simulink model "vippattern"  (R2015b)
settings: Solver=FixedStepDiscrete  SolverMode=SingleTasking  StartTime=0.0  StopTime=inf  RelTol=1e-3
InitFcn:
  | % load and initialize the data required by vippattern demo
  | 
  | % get path to the model
  | param_path = 'vippattern/Parameters';
  | 
  | % NOTE:  to set a new target run this command from command prompt:
  | % set_param(param_path,'target',mat2str(target_img))
  | % here, target_img must be a uint8 image
  | 
  | % get AVI file name straight from From MM File block
  | fmmf_path = 'vippattern/From Multimedia File';
  | 
  | % get target which is stored in a hidden parameter of 'Edit Parameters'
  | % subsystem
  | target_img = uint8(eval(get_param(param_path,'target')));
  | 
  | % Create a pyramiding factor variable and initialize it.
  | % Set the pyramiding factor by grabbing it from the masked block
  | % called 'Edit Parameters'
  | pfactor = str2double(get_param(param_path,'pfactor'));
  | 
  | target_dim_nopyramid = size(target_img);
  | % dims for gaussian pyramid
  | target_dim = ceil(target_dim_nopyramid/(2^pfactor));
  | video_info = dspmmfileinfo(get_param(fmmf_path,'inputFilename'));
  | iut_dim = ceil([video_info.videoHeightInPixels video_info.videoWidthInPixels]/2^(pfactor));
  | 
  | % figure out the sizes after padding; padding is necessary in order
  | % to avoid circular convolution
  | target_pad_rows = 2^nextpow2(iut_dim(1)+target_dim(1)+1);
  | target_pad_cols = 2^nextpow2(iut_dim(2)+target_dim(2)+1);
  | 
  | % number of targets to detect (targets are assumed to be identical)
  | num_targets = str2double(get_param(param_path,'num_targets'));
undefined symbols (not defined in the file or in its folder): gray, hot
libraries: visiontransforms x5, visionsinks x3, visionutilities x2, visionstatistics x2, dspvision x1, visiontextngfix x1, vipmisc x1, visiongeotforms x1, visionfilter x1
CloseFcn:
  | clear video_info;
  | clear iut_dim;
  | clear param_path;
  | clear fmmf_path;
  | clear pfactor;
  | clear target_dim;
  | clear target_dim_nopyramid;
  | clear target_img;
  | clear target_pad_cols;
  | clear target_pad_rows;
  | clear num_targets;
settings Model: FPTRunName=Active  ExtModeAutoUpdateStatusClock=off  Creator=The MathWorks, Inc.  LastModifiedBy=The MathWorks, Inc.
settings DataIOCC: LimitDataPoints=off  SaveFormat=Array  SaveOutput=off  SignalLogging=off  SaveTime=off  SignalLoggingName=sigsOut
settings OptimizationCC: ExpressionDepthLimit=2147483647  InitFltsAndDblsToZero=on  EfficientMapNaN2IntZero=off
settings DebuggingCC: UnderspecifiedInitializationDetection=Classic  MergeDetectMultiDrivingBlocksExec=none  CheckExecutionContextPreStartOutputMsg=on  CheckExecutionContextRuntimeOutputMsg=on  SignalResolutionControl=TryResolveAllWithWarning  InheritedTsInSrcMsg=none  MultiTaskDSMMsg=warning  MultiTaskCondExecSysMsg=none  FcnCallInpInsideContextMsg=UseLocalSettings  StateNameClashWarn=warning
settings HardwareCC: ProdBitPerPointer=32  ProdLargestAtomicFloat=None  ProdIntDivRoundTo=Undefined  ProdEndianess=Unspecified  ProdWordSize=32  ProdHWDeviceType=Specified  TargetBitPerLong=64  TargetBitPerPointer=64  TargetLongLongMode=on  TargetIntDivRoundTo=Zero  TargetEndianess=LittleEndian  TargetWordSize=64  TargetHWDeviceType=Generic->MATLAB Host Computer  ProdEqTarget=off
settings ModelReferenceCC: UpdateModelReferenceTargets=IfOutOfDate
settings SFSimCC: SFSimEcho=off  SimParseCustomCode=off
settings GRTTargetCC: TargetFcnLib=ansi_tfl_tmw_new.mat  GeneratePreprocessorConditionals=Disable all  CombineOutputUpdateFcns=off  GRTInterface=on
settings ConfigComp: CovModelRefEnable=Off

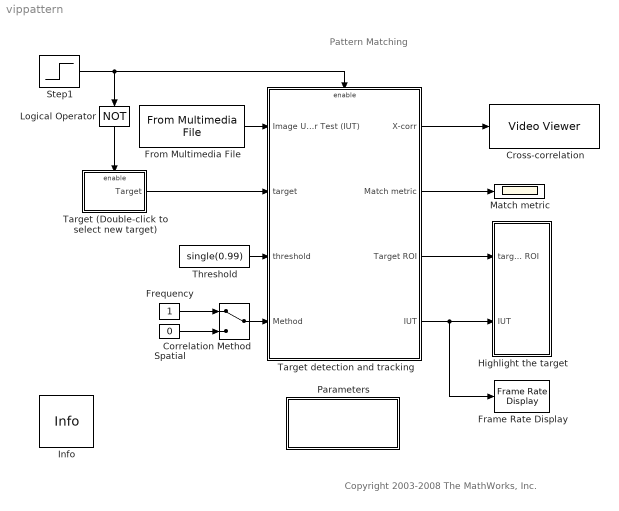
== system vippattern ==
  note: Pattern Matching
  note: Copyright 2003-2008 The MathWorks, Inc.
  Correlation Method : ManualSwitch
  Cross-correlation : visionsinks/Video Viewer  inputType=Obsolete7b  imagePorts=One multidimensional signal  useColorMap=on  colormapValue=hot(256)  specRange=on  minInputVal=0.9  maxInputVal=0.999  FigPos=[632 384 339 256]  AxisZoom=on  trueSizedOnce=off  OpenAtMdlStart=on  DefaultConfigurationName=vipscopes.VideoViewerScopeCfg
  Frame Rate Display : visionsinks/Frame Rate Display  UpdateRate=10
  Frequency : Constant  VectorParams1D=off
  From Multimedia File : dspvision/From Multimedia File  inputFilename=vipboard.avi  loop=on  numPlays=inf  outputStreams=Video and audio  videoDataType=single  audioDataType=int16  inheritSampleTime=on  userDefinedSampleTime=1/30  noAudioOutput=off  isIntensityVideo=off  fourcc=Intensity  colorVideoFormat=Separate color signals  outputEOF=off  dataOrg=Column-major  audioFrameSize=1024  computeAudioFrameSize=off  outSamplingMode=Frame based
  Highlight the target : Subsystem
  Info : vipmisc/Info  SystemSampleTime=-1
  Logical Operator : Logic  Operator=NOT  AllPortsSameDT=off  OutDataTypeStr=boolean
  Match metric : Scope
  Parameters : Subsystem  mask(Pyramiding factor){pfactor=2, num_targets=2, target=[98 98 97 98 107 108 108 108 114 115 115 115 107 105 133 177 205 204 221 184 150 155 165 172 184 178 170 162 156 191 196 222 179 136 97 109 151 175 147 147 210 241 199 180 146 128 108 96 148 183 209 223 224 189 155 151 167 171 143 145 149 127 127 154 183 197 212;99 98 98 99 106 107 107 107 114 114 114 114 105 103 130 170 164 143 152 129 119 123 131 139 137 130 122 117 134 153 129 139 133 117 94 118 110 122 118 123 147 141 163 141 123 121 116 110 115 130 138 147 154 128 123 137 127 138 107 116 108 123 116 99 123 122 136;107 107 107 108 111 111 111 111 119 119 119 119 111 109 110 112 110 103 106 112 108 110 113 108 112 109 109 112 116 110 108 105 117 118 119 107 108 113 112 111 112 112 118 115 117 118 121 120 112 106 104 121 111 100 107 116 121 121 121 117 106 109 119 114 106 105 102;108 108 108 108 113 113 113 113 114 113 113 114 122 122 122 120 114 114 114 114 112 111 111 111 111 111 112 112 111 112 112 112 108 107 109 118 118 116 118 127 120 119 118 119 117 117 117 116 116 118 114 117 125 122 120 120 119 118 119 119 118 115 111 109 109 110 110;108 108 108 108 102 101 101 102 109 110 109 111 126 127 127 126 118 117 117 116 116 115 116 115 115 115 116 116 116 116 117 116 112 111 113 122 108 107 108 112 122 123 123 123 121 120 121 120 111 119 127 127 137 137 135 134 123 123 123 124 129 120 106 98 109 110 110;107 107 107 110 147 150 148 151 173 175 174 172 182 183 184 183 180 180 182 183 176 175 176 176 177 177 175 176 179 180 179 180 183 184 183 176 185 186 186 184 186 186 186 186 181 181 182 181 170 172 175 175 184 184 182 182 187 187 188 185 136 120 104 93 108 110 110;98 99 101 106 144 147 146 147 135 158 173 149 154 142 142 143 129 126 139 149 124 121 122 123 120 121 122 122 120 118 114 115 130 131 131 130 139 140 140 139 135 133 133 132 130 131 132 131 124 123 123 122 122 122 122 122 126 125 126 123 97 98 106 109 100 104 112;104 102 98 95 80 78 78 80 96 96 95 98 80 76 76 77 71 72 63 56 74 76 75 76 74 75 75 75 76 75 75 74 70 70 70 71 75 75 76 75 65 68 71 72 82 81 78 78 65 63 64 64 64 64 64 64 76 76 76 76 85 92 101 106 99 104 112;115 107 94 85 77 76 76 75 71 80 98 109 84 82 84 83 77 76 78 79 80 80 80 80 81 80 80 80 80 80 79 80 84 85 85 84 82 82 81 82 90 89 88 88 77 78 81 80 78 78 78 78 77 77 77 78 83 83 83 82 78 83 92 97 98 104 112;121 110 90 77 77 79 80 82 71 72 80 83 82 83 84 82 68 67 70 72 79 80 80 80 81 80 80 80 80 80 79 80 82 82 82 81 72 71 71 72 86 86 86 86 89 89 89 88 74 72 72 75 77 76 76 76 74 73 73 72 76 80 87 94 99 105 113;116 105 85 71 65 68 74 79 75 77 81 77 76 76 78 78 76 75 79 82 80 80 80 81 81 81 80 80 81 80 79 80 81 81 81 81 82 83 82 82 83 82 81 81 83 84 85 84 80 79 80 79 77 78 77 78 80 77 75 72 80 103 114 106 114 116 116;113 106 93 84 81 81 82 84 82 68 68 67 73 70 83 82 81 81 83 85 86 87 87 87 85 86 87 87 87 84 80 81 86 86 86 86 84 84 84 84 84 84 84 84 84 81 78 79 85 86 86 82 78 79 79 79 77 79 83 82 70 99 121 118 116 117 116;111 110 106 101 71 73 79 85 93 76 76 87 80 79 83 83 89 90 88 85 87 87 87 88 85 86 87 87 87 87 85 86 86 86 86 86 84 84 84 84 83 84 86 85 86 83 80 81 85 85 85 85 85 85 86 85 75 82 94 102 115 135 136 119 115 116 116;109 112 115 124 166 135 89 67 92 95 90 101 83 84 82 83 93 95 89 84 87 87 87 87 85 86 87 87 86 89 92 91 86 85 85 85 84 83 84 83 83 84 86 86 86 85 85 85 84 84 83 87 91 90 91 89 73 86 108 122 185 183 150 115 114 117 116;102 104 129 170 212 157 99 82 86 88 83 83 84 85 85 85 83 82 82 82 85 86 86 86 85 85 85 85 85 85 86 85 83 83 83 83 83 83 83 83 85 86 86 86 85 85 85 84 78 78 78 78 80 80 80 80 78 82 117 157 150 169 159 122 116 117 117;104 101 122 156 183 174 126 76 78 81 82 82 85 85 85 85 81 81 81 82 85 86 86 86 85 85 85 85 85 84 84 84 83 82 83 83 83 83 83 83 86 86 86 86 85 85 85 84 82 82 82 82 83 83 83 83 79 79 109 149 168 164 140 114 116 118 118;106 98 109 136 156 155 116 70 79 82 82 82 85 85 85 85 82 81 81 82 85 86 86 86 84 84 84 84 85 85 85 84 82 82 82 82 83 83 82 83 85 85 85 85 85 85 84 85 88 88 88 88 89 89 90 89 81 76 95 131 145 124 108 110 117 118 118;108 96 100 123 137 99 69 71 ...(+5502 chars)], targetBBox=[17 99 66.0000000000001 40]}
      mask prompts: pfactor "Pyramiding factor:"; num_targets "Number of similar targets to detect:"; targetBBox "Target bounding box:"
      mask help: The pyramiding factor is used to scale the input video so that the cross-correlation is performed on a much smaller video frame thus speeding up the pattern matching process. The factor can be any number from 1 to 5. The accuracy of the match will degrade proportionately to the size of the pyramiding factor.
      mask init:
      | if num_targets <= 0
      |     error('Number of targets must be greater than 0');
      | end
      mask TypeOptions pfactor: 0 | 1 | 2 | 3 | 4 | 5
      mask Display: disp('Edit\nParameters')
  Spatial : Constant  Value=0  VectorParams1D=off
  Step1 : Step  Time=eps
  Target (Double-click to select new target) : Subsystem
      mask init:
      | model_path = [get(bdroot(gcbh),'Path'), '/Parameters'];
      | target_img = uint8(eval(get_param(model_path,'target')));
      settings: OpenFcn=vippattern_gettemplate
      mask Display: image(repmat(target_img,[1,1,3]))
  Target detection and tracking : Subsystem
  Threshold : Constant  Value=single(0.99)  VectorParams1D=off
  wires:
  From Multimedia File/1 -> Target detection and tracking/1(Image Under Test (IUT))
  Target (Double-click to select new target)/1(Target) -> Target detection and tracking/2(target)
  Target detection and tracking/1(X-corr) -> Cross-correlation/1
  Target detection and tracking/2(Match metric) -> Match metric/1
  Threshold/1 -> Target detection and tracking/3(threshold)
  Target detection and tracking/3(Target ROI) -> Highlight the target/1(target ROI)
  Target detection and tracking/4(IUT) -> Highlight the target/2(IUT), Frame Rate Display/1
  Spatial/1 -> Correlation Method/2
  Frequency/1 -> Correlation Method/1
  Correlation Method/1 -> Target detection and tracking/4(Method)
  Step1/1 -> Target detection and tracking/Enable, Logical Operator/1
  Logical Operator/1 -> Target (Double-click to select new target)/Enable

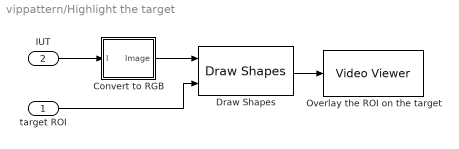
== system vippattern/Highlight the target ==
  target ROI : Inport
  IUT : Inport  Port=2
  Convert to RGB : Subsystem
  Draw Shapes : visiontextngfix/Draw Shapes  shape=Rectangles  fill=off  lineWidth=1  fillClrSource=Specify via dialog  display=User-specified value  intensity=200  color=[0 255 0]  opacity=0.6  viewport=Entire image  antialiasing=off  inType=Obsolete  imagePorts=One multidimensional signal  prodOutputMode=Binary point scaling  prodOutputWordLength=32  prodOutputFracLength=14  memoryMode=Specify word length  memoryWordLength=16  memoryFracLength=15  roundingMode=Floor  overflowMode=off
  Overlay the ROI on the target : visionsinks/Video Viewer  inputType=Obsolete7b  imagePorts=One multidimensional signal  useColorMap=off  colormapValue=gray(256)  specRange=off  minInputVal=0  maxInputVal=255  FigPos=[255 386 360 262]  AxisZoom=on  trueSizedOnce=on  OpenAtMdlStart=on  DefaultConfigurationName=vipscopes.VideoViewerScopeCfg
  wires:
  Draw Shapes/1 -> Overlay the ROI on the target/1
  target ROI/1 -> Draw Shapes/2
  Convert to RGB/1(Image) -> Draw Shapes/1
  IUT/1 -> Convert to RGB/1(I)

== system vippattern/Parameters ==

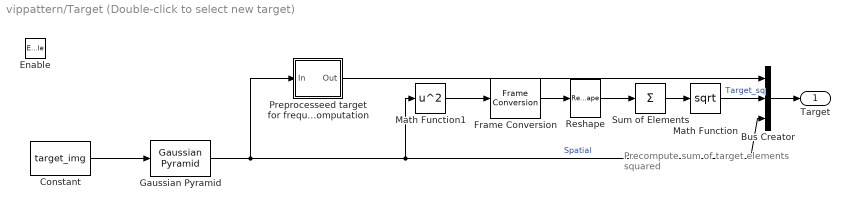
== system vippattern/Target (Double-click to select new target) ==
  note: Precompute sum of target elements
      | squared
  Enable : EnablePort  PropagateVarSize=During execution
  Bus Creator : BusCreator  Inputs=3
  Constant : Constant  Value=target_img  VectorParams1D=off  OutDataTypeStr=single
  Frame Conversion : FrameConversion  InheritSamplingMode=off  OutFrame=Sample-based
  Gaussian Pyramid : visiontransforms/Gaussian Pyramid  operation=Reduce  level=pfactor  source="Default separable filter [1/4-a/2  1/4  a  1/4  1/4-a/2]"  a=0.375  coef=[0.0625 0.25 0.375 0.25 0.0625]  hiddenCoef=[1/4-0.375/2 1/4 0.375 1/4 1/4-0.375/2]  firstCoeffMode=Specify word length  firstCoeffWordLength=16  firstCoeffFracLength=16  outputMode=Binary point scaling  outputWordLength=32  outputFracLength=10  prodOutputMode=Binary point scaling  prodOutputWordLength=32  prodOutputFracLength=10  roundingMode=Floor  overflowMode=off
  Math Function : Math  Operator=sqrt  SaturateOnIntegerOverflow=on
  Math Function1 : Math  Operator=square  SaturateOnIntegerOverflow=on
  Preprocesseed target for frequency domain computation : Subsystem
  Reshape : Reshape
  Sum of Elements : Sum  Inputs=+
  Target : Outport
  wires:
  Preprocesseed target for frequency domain computation/1(Out) -> Bus Creator/1
  Bus Creator/1 -> Target/1
  Constant/1 -> Gaussian Pyramid/1
  Gaussian Pyramid/1 -> Preprocesseed target for frequency domain computation/1(In), Bus Creator/3, Math Function1/1  "Spatial"
  Math Function1/1 -> Frame Conversion/1
  Sum of Elements/1 -> Math Function/1
  Reshape/1 -> Sum of Elements/1
  Math Function/1 -> Bus Creator/2  "Target_sq"
  Frame Conversion/1 -> Reshape/1

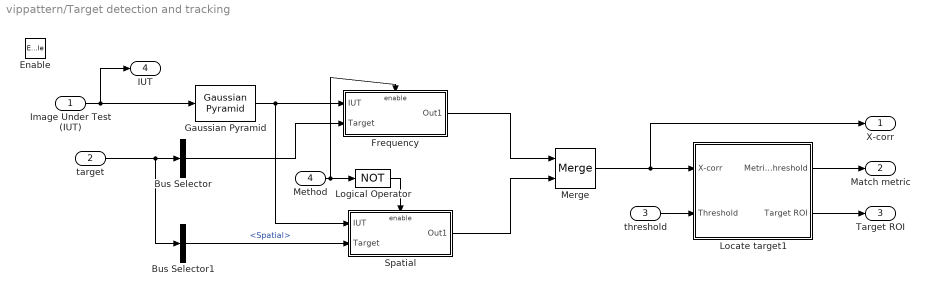
== system vippattern/Target detection and tracking ==
  Image Under Test (IUT) : Inport
  target : Inport  Port=2
  threshold : Inport  Port=3
  Method : Inport  Port=4
  Enable : EnablePort  PropagateVarSize=During execution
  Bus Selector : BusSelector  OutputSignals=Frequency,Target_sq  OutputAsBus=on
  Bus Selector1 : BusSelector  OutputSignals=Spatial
  Frequency : Subsystem  TreatAsAtomicUnit=on
  Gaussian Pyramid : visiontransforms/Gaussian Pyramid  operation=Reduce  level=pfactor  source="Default separable filter [1/4-a/2  1/4  a  1/4  1/4-a/2]"  a=0.375  coef=[0.0625 0.25 0.375 0.25 0.0625]  hiddenCoef=[1/4-0.375/2 1/4 0.375 1/4 1/4-0.375/2]  firstCoeffMode=Specify word length  firstCoeffWordLength=16  firstCoeffFracLength=16  outputMode=Binary point scaling  outputWordLength=32  outputFracLength=10  prodOutputMode=Binary point scaling  prodOutputWordLength=32  prodOutputFracLength=10  roundingMode=Floor  overflowMode=off
  Locate target1 : Subsystem
  Logical Operator : Logic  Operator=NOT  AllPortsSameDT=off  OutDataTypeStr=boolean
  Merge : Merge
  Spatial : Subsystem  TreatAsAtomicUnit=on
  X-corr : Outport
  Match metric : Outport  Port=2
  Target ROI : Outport  Port=3
  IUT : Outport  Port=4
  wires:
  Image Under Test (IUT)/1 -> IUT/1, Gaussian Pyramid/1
  Locate target1/1(Metric and Threshold) -> Match metric/1
  threshold/1 -> Locate target1/2(Threshold)
  Gaussian Pyramid/1 -> Frequency/1(IUT), Spatial/1(IUT)
  target/1 -> Bus Selector/1, Bus Selector1/1
  Bus Selector/1 -> Frequency/2(Target)
  Bus Selector1/1 -> Spatial/2(Target)  "<Spatial>"
  Spatial/1(Out1) -> Merge/2
  Merge/1 -> X-corr/1, Locate target1/1(X-corr)
  Frequency/1(Out1) -> Merge/1
  Logical Operator/1 -> Spatial/Enable
  Method/1 -> Logical Operator/1, Frequency/Enable
  Locate target1/2(Target ROI) -> Target ROI/1

== system vippattern/Highlight the target/Convert to RGB ==
  I : Inport
  Matrix Concatenate : Concatenate  NumInputs=3  Mode=Multidimensional array  ConcatenateDimension=3
  Image : Outport
  wires:
  I/1 -> Matrix Concatenate/1, Matrix Concatenate/2, Matrix Concatenate/3
  Matrix Concatenate/1 -> Image/1

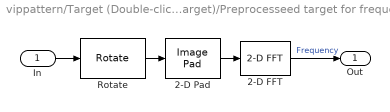
== system vippattern/Target (Double-click to select new target)/Preprocesseed target for frequency domain computation ==
  In : Inport
  2-D FFT : visiontransforms/2-D FFT  TableOpt=NEW  TableOptActive=Speed  BitRevOrder=off  SkipNorm=off  FFTImplementation=Auto  firstCoeffDataTypeStr=Inherit: Same word length as input  firstCoeffLastDataTypeStr=Inherit: Same word length as input  outputMin=[]  outputMax=[]  accumDataTypeStr=Inherit: Same as product output  accumLastDataTypeStr=Inherit: Same as product output  roundingMode=Floor  overflowMode=off
  2-D Pad : visionutilities/Image Pad  method=Constant  valSrc=Specify via dialog  value=0  spec=Output size  rowDirection=Right  outRowsMode=User-specified  rowSize=2  outColSize=2^nextpow2(iut_dim(2)+target_dim(2)+1)  colDirection=Bottom  outColsMode=User-specified  colSize=[2 3]  outRowSize=2^nextpow2(iut_dim(1)+target_dim(1)+1)  trunc_flag=None
  Rotate : visiongeotforms/Rotate  outSizeR=Expanded to fit rotated input image  src_angle=Specify via dialog  unit_angle=Degrees  angle=single(pi)  maxAngle=pi  dispImage=Center  method=Table lookup  fillVal=0  interpMethod=Bilinear  prodOutputMode=Binary point scaling  prodOutputWordLength=32  prodOutputFracLength=10  roundingMode=Nearest  overflowMode=on
  Out : Outport
  wires:
  Rotate/1 -> 2-D Pad/1
  2-D Pad/1 -> 2-D FFT/1
  In/1 -> Rotate/1
  2-D FFT/1 -> Out/1  "Frequency"

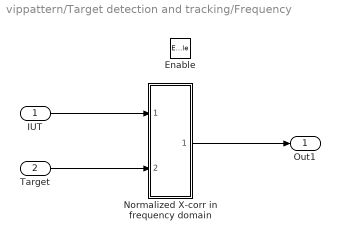
== system vippattern/Target detection and tracking/Frequency ==
  IUT : Inport
  Target : Inport  Port=2
  Enable : EnablePort  PropagateVarSize=During execution
  Normalized X-corr in frequency domain : Subsystem
  Out1 : Outport  InitialOutput=0
  wires:
  Normalized X-corr in frequency domain/1(X-corr) -> Out1/1
  IUT/1 -> Normalized X-corr in frequency domain/1(IUT)
  Target/1 -> Normalized X-corr in frequency domain/2(target)

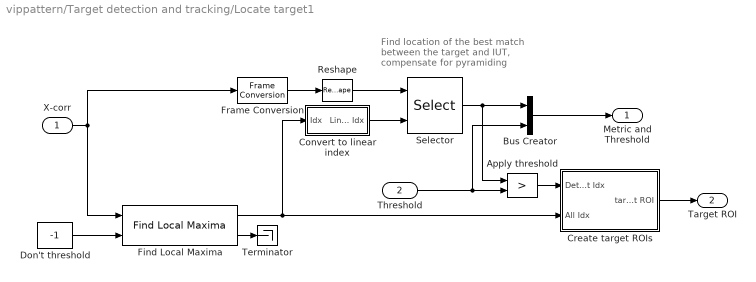
== system vippattern/Target detection and tracking/Locate target1 ==
  note: Find location of the best match
      | between the target and IUT,
      | compensate for pyramiding
  X-corr : Inport
  Threshold : Inport  Port=2
  Apply threshold : RelationalOperator  Operator=>  OutDataTypeStr=boolean  ZeroCross=off
  Bus Creator : BusCreator  Inputs=2
  Convert to linear index : Subsystem
  Create target ROIs : Subsystem
  Don't threshold : Constant  Value=-1  VectorParams1D=off  OutDataTypeStr=Inherit: Inherit via back propagation
  Find Local Maxima : visionstatistics/Find Local Maxima  num_peaks=num_targets  nhood_size=floor(target_dim/2)*2-1  src_thresh=Obsolete9b  src_thresh_inuse=Input port  threshold=10  inputIsHough=off  dt_peak=single  isOutVarDim=off  dt_count=single
  Frame Conversion : FrameConversion  InheritSamplingMode=off  OutFrame=Sample-based
  Reshape : Reshape
  Selector : Selector  IndexMode=Zero-based  InputPortWidth=prod(((iut_dim-target_dim)+1))  IndexOptions=Index vector (port)  Indices=[1 3]  OutputSizes=1
  Terminator : Terminator
  Metric and Threshold : Outport
  Target ROI : Outport  Port=2
  wires:
  Threshold/1 -> Bus Creator/2, Apply threshold/2
  Create target ROIs/1(target ROI) -> Target ROI/1
  Reshape/1 -> Selector/1
  Convert to linear index/1(Linear Idx) -> Selector/2
  Bus Creator/1 -> Metric and Threshold/1
  Apply threshold/1 -> Create target ROIs/1(Detected-target Idx)
  Don't threshold/1 -> Find Local Maxima/2
  Find Local Maxima/2 -> Terminator/1
  Selector/1 -> Bus Creator/1, Apply threshold/1
  Find Local Maxima/1 -> Create target ROIs/2(All Idx), Convert to linear index/1(Idx)
  X-corr/1 -> Find Local Maxima/1, Frame Conversion/1
  Frame Conversion/1 -> Reshape/1

== system vippattern/Target detection and tracking/Spatial ==
  IUT : Inport
  Target : Inport  Port=2
  Enable : EnablePort  PropagateVarSize=During execution
  Normalized X-corr in spatial domain : visionstatistics/2-D Correlation  outSize=Valid  normalize=on  roundingMode=Floor  overflowMode=off
  Out1 : Outport  InitialOutput=0
  wires:
  Target/1 -> Normalized X-corr in spatial domain/2
  IUT/1 -> Normalized X-corr in spatial domain/1
  Normalized X-corr in spatial domain/1 -> Out1/1

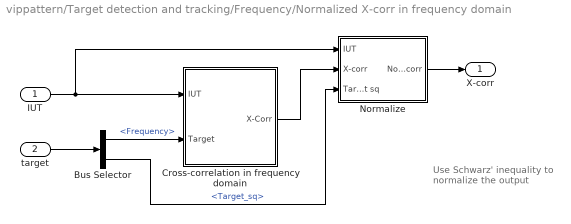
== system vippattern/Target detection and tracking/Frequency/Normalized X-corr in frequency domain ==
  note: Use Schwarz' inequality
      | to normalize the output
  IUT : Inport
  target : Inport  Port=2
  Bus Selector : BusSelector  OutputSignals=Frequency,Target_sq
  Cross-correlation in frequency domain : Subsystem
  Normalize : Subsystem
  X-corr : Outport
  wires:
  target/1 -> Bus Selector/1
  Normalize/1(Norm X-corr) -> X-corr/1
  IUT/1 -> Cross-correlation in frequency domain/1(IUT), Normalize/1(IUT)
  Cross-correlation in frequency domain/1(X-Corr) -> Normalize/2(X-corr)
  Bus Selector/1 -> Cross-correlation in frequency domain/2(Target)  "<Frequency>"
  Bus Selector/2 -> Normalize/3(Target sq)  "<Target_sq>"

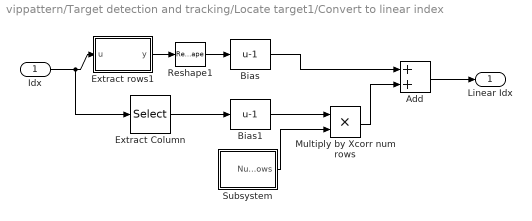
== system vippattern/Target detection and tracking/Locate target1/Convert to linear index ==
  Idx : Inport
  Add : Sum
  Bias : Bias  Bias=-1  SaturateOnIntegerOverflow=on
  Bias1 : Bias  Bias=-1  SaturateOnIntegerOverflow=on
  Extract Column : Selector  NumberOfDimensions=2  InputPortWidth=3  IndexOptions=Select all,Index vector (dialog)  Indices=[target_dim(1):iut_dim(1)],[1]  OutputSizes=1,1
  Extract rows1 : MATLAB Function  TreatAsAtomicUnit=on
  Multiply by Xcorr num rows : Product  OutDataTypeStr=uint32  RndMeth=Zero
  Reshape1 : Reshape  OutputDimensionality=Column vector (2-D)
  Subsystem : Subsystem
  Linear Idx : Outport
  wires:
  Add/1 -> Linear Idx/1
  Idx/1 -> Extract rows1/1(u), Extract Column/1
  Subsystem/1(Num Rows) -> Multiply by Xcorr num rows/2
  Extract rows1/1(y) -> Reshape1/1
  Multiply by Xcorr num rows/1 -> Add/2
  Extract Column/1 -> Bias1/1
  Bias/1 -> Add/1
  Bias1/1 -> Multiply by Xcorr num rows/1
  Reshape1/1 -> Bias/1

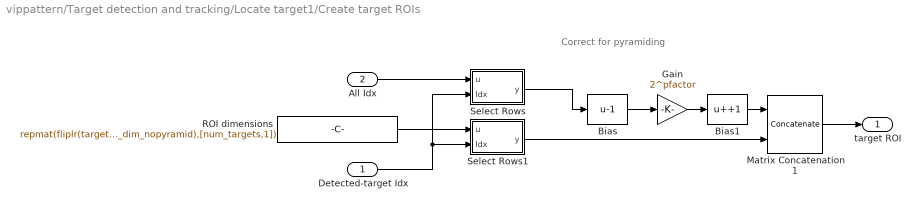
== system vippattern/Target detection and tracking/Locate target1/Create target ROIs ==
  note: Correct for
      |  pyramiding
  Detected-target Idx : Inport
  All Idx : Inport  Port=2
  Bias : Bias  Bias=-1  SaturateOnIntegerOverflow=on
  Bias1 : Bias  Bias=+1  SaturateOnIntegerOverflow=on
  Gain : Gain  Gain=2^pfactor  ParamDataTypeStr=float('single')  RndMeth=Nearest  SaturateOnIntegerOverflow=on  OutDataTypeStr=Inherit: Same as input
  Matrix Concatenation1 : Concatenate  Mode=Multidimensional array  ConcatenateDimension=2
  ROI dimensions : Constant  Value=repmat(fliplr(target_dim_nopyramid),[num_targets,1])  VectorParams1D=off  OutDataTypeStr=single
  Select Rows : MATLAB Function  TreatAsAtomicUnit=on
  Select Rows1 : MATLAB Function  TreatAsAtomicUnit=on
  target ROI : Outport
  wires:
  Detected-target Idx/1 -> Select Rows/2(Idx), Select Rows1/2(Idx)
  All Idx/1 -> Select Rows/1(u)
  Select Rows/1(y) -> Bias/1
  Matrix Concatenation1/1 -> target ROI/1
  Gain/1 -> Bias1/1
  Select Rows1/1(y) -> Matrix Concatenation1/2
  Bias/1 -> Gain/1
  Bias1/1 -> Matrix Concatenation1/1
  ROI dimensions/1 -> Select Rows1/1(u)

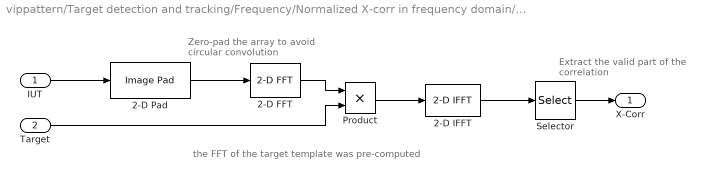
== system vippattern/Target detection and tracking/Frequency/Normalized X-corr in frequency domain/Cross-correlation in frequency domain ==
  note: Extract the valid part
      | of the correlation
  note: Zero-pad the array to avoid
      | circular convolution
  note: the FFT of the target template was pre-computed
  IUT : Inport
  Target : Inport  Port=2
  2-D FFT : visiontransforms/2-D FFT  TableOpt=NEW  TableOptActive=Speed  BitRevOrder=off  SkipNorm=off  FFTImplementation=Auto  firstCoeffDataTypeStr=Inherit: Same word length as input  firstCoeffLastDataTypeStr=Inherit: Same word length as input  outputMin=[]  outputMax=[]  accumDataTypeStr=Inherit: Same as product output  accumLastDataTypeStr=Inherit: Same as product output  roundingMode=Floor  overflowMode=off
  2-D IFFT : visiontransforms/2-D IFFT  TableOpt=HYBRID  TableOptActive=Speed  BitRevOrder=off  cs_in=on  SkipNorm=on  FFTImplementation=Auto  firstCoeffDataTypeStr=Inherit: Same word length as input  firstCoeffLastDataTypeStr=Inherit: Same word length as input  outputMin=[]  outputMax=[]  accumDataTypeStr=Inherit: Same as product output  accumLastDataTypeStr=Inherit: Same as product output  roundingMode=Floor  overflowMode=off
  2-D Pad : visionutilities/Image Pad  method=Constant  valSrc=Specify via dialog  value=0  spec=Output size  rowDirection=Right  outRowsMode=User-specified  rowSize=2  outColSize=2^nextpow2(iut_dim(2)+target_dim(2)+1)  colDirection=Bottom  outColsMode=User-specified  colSize=[2 3]  outRowSize=2^nextpow2(iut_dim(1)+target_dim(1)+1)  trunc_flag=None
  Product : Product  RndMeth=Zero
  Selector : Selector  NumberOfDimensions=2  InputPortWidth=3  IndexOptions=Index vector (dialog),Index vector (dialog)  Indices=[target_dim(1):iut_dim(1)],[target_dim(2):iut_dim(2)]  OutputSizes=1,1
  X-Corr : Outport
  wires:
  2-D Pad/1 -> 2-D FFT/1
  Target/1 -> Product/2
  IUT/1 -> 2-D Pad/1
  Selector/1 -> X-Corr/1
  2-D IFFT/1 -> Selector/1
  2-D FFT/1 -> Product/1
  Product/1 -> 2-D IFFT/1

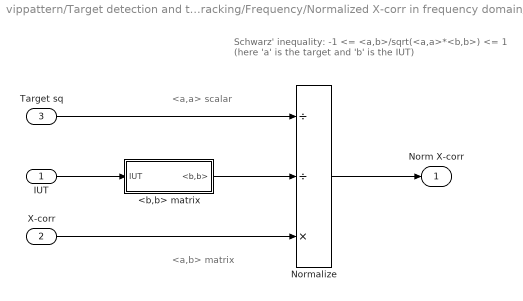
== system vippattern/Target detection and tracking/Frequency/Normalized X-corr in frequency domain/Normalize ==
  note: <a,b> matrix
  note: <a,a> scalar
  note: Schwarz' inequality:
      | -1 <= <a,b>/sqrt(<a,a>*<b,b>) <= 1
      | (here 'a' is the target and 'b' is the IUT)
  IUT : Inport
  X-corr : Inport  Port=2
  Target sq : Inport  Port=3
  <b,b> matrix : Subsystem
  Normalize : Product  Inputs=//*  SaturateOnIntegerOverflow=on  RndMeth=Zero  OutDataTypeStr=Inherit: Same as first input
  Norm X-corr : Outport
  wires:
  X-corr/1 -> Normalize/3
  Target sq/1 -> Normalize/1
  <b,b> matrix/1(<b,b>) -> Normalize/2
  Normalize/1 -> Norm X-corr/1
  IUT/1 -> <b,b> matrix/1(IUT)

== system vippattern/Target detection and tracking/Locate target1/Convert to linear index/Subsystem ==
  Selector : Selector  NumberOfDimensions=2  InputPortWidth=3  IndexOptions=Index vector (dialog),Index vector (dialog)  Indices=1,1  OutputSizes=1,1
  Xcorr dims : Constant  Value=((iut_dim-target_dim)+1)  VectorParams1D=off  OutDataTypeStr=Inherit: Inherit via back propagation
  Num Rows : Outport
  wires:
  Selector/1 -> Num Rows/1
  Xcorr dims/1 -> Selector/1

== system vippattern/Target detection and tracking/Frequency/Normalized X-corr in frequency domain/Normalize/<b,b> matrix ==
  note: use 2-D filter to
      | compute local sums
  note: Block process tiles that are the size of the target template
  IUT : Inport
  Math Function : Math  Operator=sqrt  SaturateOnIntegerOverflow=on
  Math Function1 : Math  Operator=square  SaturateOnIntegerOverflow=on
  compute local sums : visionfilter/2-D FIR Filter  separable=off  filtSrc=Specify via dialog  filterMtrx=ones(target_dim)  verticalFilter=[4 0]  horizontalFilter=[4 0]  outSize=Valid  padType=Constant  padSrc=Specify via dialog  padVal=0  method=Convolution  firstCoeffSignedness=Signed  firstCoeffDataTypeStr=Inherit: Same word length as input  firstCoeffLastDataTypeStr=Inherit: Same word length as input  firstCoeffMin=[]  firstCoeffMax=[]  outputSignedness=Auto  outputMin=[]  outputMax=[]  accumDataTypeStr=Inherit: Same as product output  accumLastDataTypeStr=Inherit: Same as product output  roundingMode=Floor  overflowMode=off
  <b,b> : Outport
  wires:
  Math Function/1 -> <b,b>/1
  Math Function1/1 -> compute local sums/1
  IUT/1 -> Math Function1/1
  compute local sums/1 -> Math Function/1

== matlab function vippattern/Target detection and tracking/Locate target1/Convert to linear index/Extract rows1 ==
  data: u input; y output
function y = fcn(u)
%#codegen
l = size(u); 
y = u(:,l(2));

== matlab function vippattern/Target detection and tracking/Locate target1/Create target ROIs/Select Rows ==
  data: u input; y output; Idx input
function y = fcn(u, Idx)
%#codegen

y = u;
y(~Idx,:)=0;

== matlab function vippattern/Target detection and tracking/Locate target1/Create target ROIs/Select Rows1 ==
  data: u input; y output; Idx input
function y = fcn(u, Idx)
%#codegen

y = u;
y(~Idx,:)=0;
